simulink model "ex8_t3"  (R2025b)
settings: Solver=ode45  StartTime=0.0  StopTime=20  RelTol=1e-3
libraries: simulink x1
settings Model: Creator=Hamidur  LastModifiedBy=Hamidur

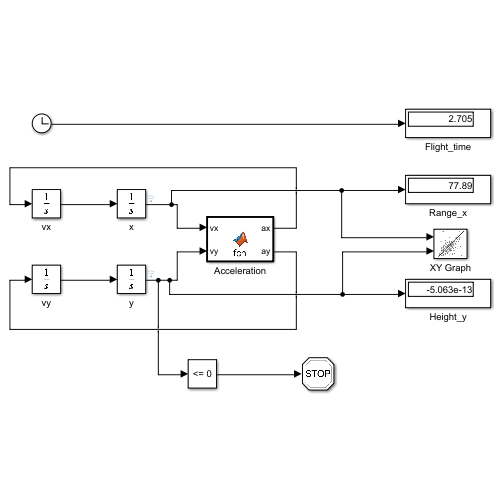
[thumbnail: Simulink's stored preview of the top-level diagram]
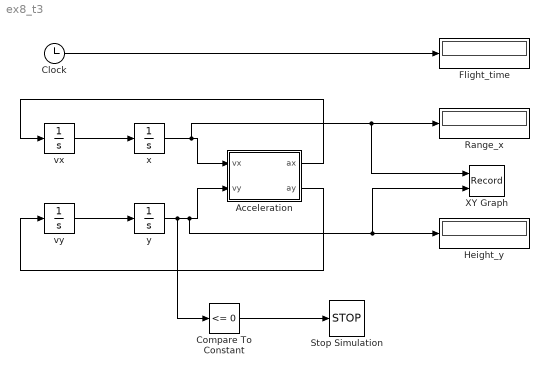
== system ex8_t3 ==
  Acceleration : MATLAB Function  TreatAsAtomicUnit=on
  Clock : Clock
  Compare To Constant : simulink/Logic and Bit Operations/Compare To Constant  relop=<=  const=0  OutDataTypeStr=boolean
  Flight_time : Display
  Height_y : Display
  Range_x : Display
  Stop Simulation : Stop
  XY Graph : Record  NumPorts=2.0  FileSettingsInternal="{\"entries\":[{\"content\":{\"excelSettings\":{\"content\":{},\"type\":\"Streamout.ExcelSettings\"},\"parquetSettings\":{\"content\":{},\"type\":\"Streamout.ParquetSettings\"}},\"type\":\"Streamout.FileSettingStorage\",\"uuid\":\"\"}],\"packageUris\":[\"http:\\/\\/schema.mathworks.com\\/mf0\\/streamout_blocks\\/R2020a\"],\"version\":\"1.0\"}"  FrameSettings=[0, 0]  Layout=[1 1]  SignalsInternal="{\"entries\":[{\"content\":{\"signals\":[{\"content\":{\"blockPath\":[],\"dimensions\":[1],\"domain\":\"\",\"lineColor\":\"#a2142f\",\"plots\":[ 1 ],\"port\":1,\"sid\":[\"\"],\"signalID\":1,\"signalName\":\"x\"},\"type\":\"RecordBlkView.Signal\",\"uuid\":\"\"},{\"content\":{\"blockPath\":[],\"dimensions\":[1],\"domain\":\"\",\"lineColor\":\"#139fff\",\"plots\":[ 1 ],\"port\":2,\"sid\":[\"\"],\"signalID\":2,\"signalName\":\"y\"},\"type\":\"RecordBlkView.Signal\",\"uuid\":\"\"}]},\"type\":\"RecordBlkView.InputSignals\",\"uuid\":\"\"}],\"packageUris\":[\"http:\\/\\/schema.mathworks.com\\/mf0\\/streamout_blocks\\/R2020a\"],\"version\":\"1.0\"}"  VisualizationBindings="{\"xyplotplugin\":{\"info\":[{\"series\":[{\"bindingParametersList\":[{\"parameter\":\"X-Axis\",\"signalID\":1,\"signalName\":\"x\"},{\"parameter\":\"Y-Axis\",\"signalID\":2,\"signalName\":\"y\"}],\"seriesID\":0}],\"subplotID\":1}]}}"  CompatibilityTag=XY
  vx : Integrator  InitialCondition=42.2862
  vy : Integrator  InitialCondition=15.3909
  x : Integrator
  y : Integrator  InitialCondition=2
  wires:
  Acceleration/1(ax) -> vx/1
  Acceleration/2(ay) -> vy/1
  vx/1 -> x/1
  x/1 -> XY Graph/1, Range_x/1, Acceleration/1(vx)
  vy/1 -> y/1
  y/1 -> Compare To Constant/1, XY Graph/2, Height_y/1, Acceleration/2(vy)
  Compare To Constant/1 -> Stop Simulation/1
  Clock/1 -> Flight_time/1

== matlab function ex8_t3/Acceleration ==
  data: vx input; ax output; vy input; ay output
function [ax, ay] = fcn(vx, vy)
m = 0.145;
rho = 1.204;
Cd = 0.3;
d = 0.075;
g = 9.81;

A = pi*(d/2)^2;

k = 0.5*rho*Cd*A;

v = sqrt(vx^2 + vy^2);

ax = -(k/m)*v*vx;
ay = -g -(k/m)*v*vy;
